simulink model "pv_array"  (R2024b)
settings: Solver=FixedStepAuto  StartTime=0.0  StopTime=10.0  FixedStep=5e-6  RelTol=1e-3
libraries: spsGroundLib x4, spsSeriesRLCBranchLib x3, spsStairGeneratorLib x2, spsBoostConverterLib x1, spsPVArrayLib x1, spsPWMGeneratorDCDCLib x1, spsVariableResistorLib x1, spsVoltageMeasurementLib x1, sps_lib x1
settings Model: LastModifiedBy=HP

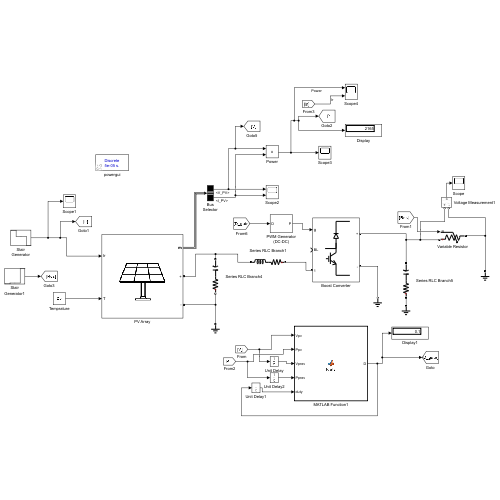
[thumbnail: Simulink's stored preview of the top-level diagram]
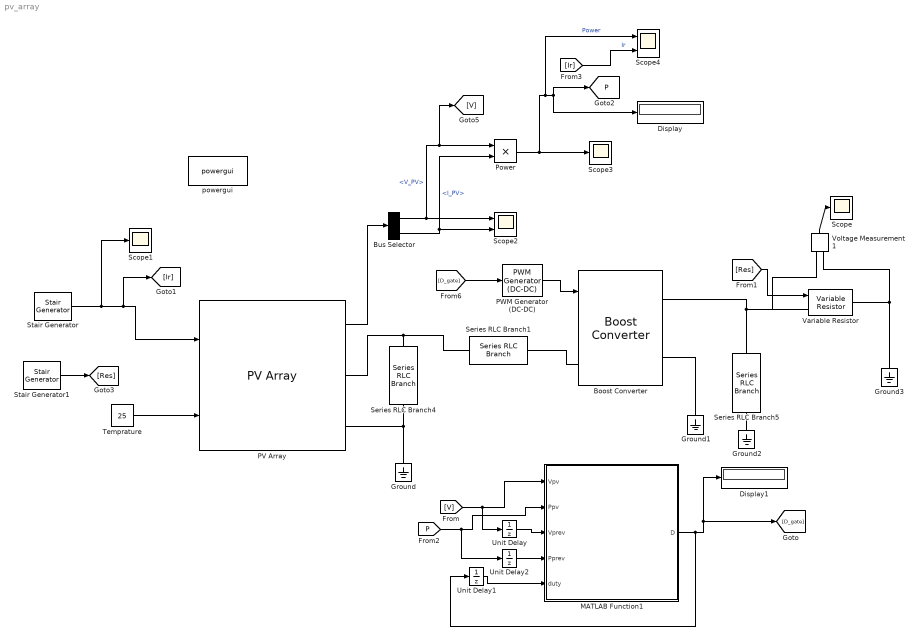
== system pv_array ==
  Boost Converter : spsBoostConverterLib/Boost Converter  ModelType=Switching devices  Ron=1e-3  Rs=1e6  Cs=inf  Vforward=[0,0]  Ron_Diode=1e-3  Rs_Diode=1e6  Cs_Diode=inf  Vf_Diode=1e-3  Rs_CurrentSource=inf  Ron_ACsource=1e-3
      settings: LibrarySourceBlock=sps_lib/Power Electronics/Boost Converter
  Bus Selector : BusSelector  OutputSignals=V_PV,I_PV
  Display : Display
  Display1 : Display
  Ground{,1..3} (4 alike) : spsGroundLib/Ground  LConnTagsString=a
  MATLAB Function1 : MATLAB Function  TreatAsAtomicUnit=on
  PV Array : spsPVArrayLib/PV Array  Npar=2  Nser=10  PlotType=array @ 25 deg.C & specified irradiances  S_vec="[ 1000  800  500 ]"  Temp_C_vec="[ 45 25  ]"  ModuleName=User-defined  PlotWhenSelected=off  Pm=213.15  Ncell=60  Voc=36.3  Isc=7.84  Vm=29  Im=7.35  beta_Voc_pc=-0.36099  alpha_Isc_pc=0.061743  beta_Voc=-0.13104  alpha_Isc=0.0048407  IL=7.8592  I0=2.7553e-10  nI=0.97871  Rsh=338.6159  Rs=0.39498  RobustModel=off  RobustCellTemperature=313.3991  BAL=on  Tc=1e-6  Tfilter=5e-5
  PWM Generator (DC-DC) : spsPWMGeneratorDCDCLib/PWM Generator (DC-DC)  Fsw=5000  Ts=0
  Power : Product
  Scope : Scope
  Scope1 : Scope
  Scope2 : Scope  NumInputPorts=2
  Scope3 : Scope
  Scope4 : Scope  NumInputPorts=2
  Series RLC Branch1 : spsSeriesRLCBranchLib/Series RLC Branch  LConnTagsString=__new0  RConnTagsString=__new0  BranchType=RL  Resistance=1e-3  Inductance=560e-6  SetiL0=off  InitialCurrent=0  Capacitance=270e-6  Setx0=off  InitialVoltage=0  Measurements=None
  Series RLC Branch4 : spsSeriesRLCBranchLib/Series RLC Branch  LConnTagsString=__new0  RConnTagsString=__new0  BranchType=RC  Resistance=1e-3  Inductance=5e-3  SetiL0=off  InitialCurrent=0  Capacitance=270e-6  Setx0=off  InitialVoltage=0  Measurements=None
  Series RLC Branch5 : spsSeriesRLCBranchLib/Series RLC Branch  LConnTagsString=__new0  RConnTagsString=__new0  BranchType=RC  Resistance=1e-3  Inductance=5e-3  SetiL0=off  InitialCurrent=0  Capacitance=4700e-6  Setx0=off  InitialVoltage=0  Measurements=None
  Stair Generator : spsStairGeneratorLib/Stair Generator  t=[0, 1, 2,3,4,5]  e=[1000,1000,800,800,500,500]  Ts=0
  Stair Generator1 : spsStairGeneratorLib/Stair Generator  t=[0, 1, 2,3,4,5]  e=[40,40,50,50,250,250]  Ts=0
  Temprature : Constant  Value=25
  Unit Delay : UnitDelay  SampleTime=-1  HasFrameUpgradeWarning=on
  Unit Delay1 : UnitDelay  SampleTime=-1  HasFrameUpgradeWarning=on
  Unit Delay2 : UnitDelay  SampleTime=-1  HasFrameUpgradeWarning=on
  Variable Resistor : spsVariableResistorLib/Variable Resistor  Rabsmin=1e-3
      settings: LibrarySourceBlock=sps_lib/Passives/Variable Resistor
  Voltage Measurement1 : spsVoltageMeasurementLib/Voltage Measurement  PhasorSimulation=off  OutputType=Complex  PSBequivalent=0
  powergui : sps_lib/powergui  Priority=1  SimulationMode=Discrete  SampleTime=5e-5  frequency=60  Iterations=50  frequencyindice=0  Pbase=100e6  ErrMax=1e-4  UnitsV=kV  UnitsW=MW  buscounter=0  FunctionMessages=off  echomessages=off  EnableUseOfTLC=off  CurrentSourceSwitches=off  DisableSnubberDevices=off  DisableRonSwitches=off  DisableVfSwitches=off  DisplayEquations=off  AutomaticDiscreteSolvers=off  SolverType=Tustin/Backward Euler (TBE)  Interpol=off  ExternalGateDelay=off  methode=off  Ts=100  x0status=blocks  SPID=on  SwTol=0  HookPort=off  NonlinearTolerance=1e-4  nMaxIteration=100  ContinueOnMaxIteration=off  RestoreLinks=warning  ResistiveCurrentMeasurement=off  Frange=[0:2:500]  Ylog=off  Xlog=on  ShowGrid=off  save=off  variable=ZData  structure=0  ZoomFFT=off  StartTime=0.0  cycles=1  DisplayStyle=1  fundamental=60  FreqAxis=off  MaxFrequency=1000  frequencyindicesteady=1  RmsSteady=1  display=off
  tag scope: P=global
  wires:
  PV Array/1 -> Bus Selector/1
  Stair Generator/1 -> Scope1/1, [Ir], PV Array/1
  Temprature/1 -> PV Array/2
  Power/1 -> Scope4/1, [P], Display/1, Scope3/1  "Power"
  Bus Selector/1 -> [V], Power/1, Scope2/1  "<V_PV>"
  Bus Selector/2 -> Power/2, Scope2/2  "<I_PV>"
  PWM Generator (DC-DC)/1 -> Boost Converter/1
  [D_gate] -> PWM Generator (DC-DC)/1
  Voltage Measurement1/1 -> Scope/1
  Stair Generator1/1 -> [Res]
  [V] -> MATLAB Function1/1(Vpv), Unit Delay/1
  Unit Delay1/1 -> MATLAB Function1/5(duty)
  MATLAB Function1/1(D) -> Display1/1, [D_gate], Unit Delay1/1
  Unit Delay/1 -> MATLAB Function1/3(Vprev)
  [P] -> MATLAB Function1/2(Ppv), Unit Delay2/1
  Unit Delay2/1 -> MATLAB Function1/4(Pprev)
  [Ir] -> Scope4/2  "Ir"
  [Res] -> Variable Resistor/1
  connections:
  PV Array/RConn1 -- Series RLC Branch1/RConn1 -- Series RLC Branch4/RConn1
  Ground/LConn1 -- Series RLC Branch4/LConn1 -- PV Array/RConn2
  Series RLC Branch1/LConn1 -- Boost Converter/LConn1
  Boost Converter/RConn2 -- Ground1/LConn1
  Boost Converter/RConn1 -- Variable Resistor/LConn1 -- Voltage Measurement1/LConn1 -- Series RLC Branch5/RConn1
  Ground2/LConn1 -- Series RLC Branch5/LConn1
  Voltage Measurement1/LConn2 -- Ground3/LConn1 -- Variable Resistor/RConn1

== matlab function pv_array/MATLAB Function1 ==
  data: Vpv input; D output; Ppv input; Vprev input; Pprev input; duty input
function D = fduty (Vpv, Ppv, Vprev, Pprev, duty)
dD=0.001;
Dmin=0.1;
Dmax=0.95;
if isempty(duty)
     duty=0.5;
end
dP=Ppv-Pprev;
dV=Vpv-Vprev;

if dP>0
  if dV>0
     D=duty-dD;
  else
     D=duty+dD;
  end
else
    if dV>0
      D=duty+dD;
    else
       D=duty-dD;
    end
end   
D= max(min(D,Dmax),Dmin);
